simulink model "VelocityTransitionHandler"  (R2016b)
settings: Solver=FixedStepAuto  StartTime=0.0  StopTime=10.0  FixedStep=0.002  RelTol=1e-3  EnableMultiTasking=on
settings Model: Creator=march  LastModifiedBy=snyke7
settings SolverCC: EnableConcurrentExecution=on
settings DataIOCC: SaveFormat=StructureWithTime
settings OptimizationCC: BlockReduction=off  OptimizeBlockIOStorage=off  BufferReuse=off  GlobalBufferReuse=off  ExpressionFolding=off  LocalBlockOutputs=off
settings HardwareCC: ProdBitPerPointer=32  ProdBitPerSizeT=32  ProdBitPerPtrDiffT=32  ProdLargestAtomicFloat=None  ProdWordSize=32  ProdLongLongMode=on  ProdHWDeviceType=Generic->32-bit x86 compatible
settings RTWCC: SystemTargetFile=slrt.tlc  TemplateMakefile=slrt_default_tmf  Description=Simulink Real-Time  RTWCompilerOptimization=on
settings TargetCC: CodeReplacementLibrary=XPC_BLAS  ParMdlRefBuildCompliant=on  ConcurrentExecutionCompliant=on  GeneratePreprocessorConditionals=Use local settings  MatFileLogging=on  MATLABClassNameForMDSCustomization=xpcAperiodicCustomization

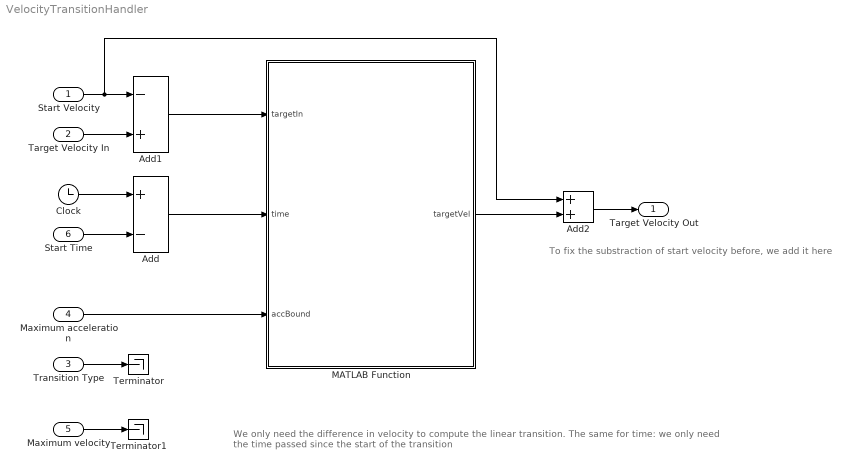
== system VelocityTransitionHandler ==
  note: To fix the substraction of start velocity before, we add it here
  note: We only need the difference in velocity to compute the linear transition. The same for time: we only need the time passed since the start of the transition
  Start Velocity : Inport
  Target Velocity In : Inport  Port=2
  Transition Type : Inport  Port=3
  Maximum acceleration : Inport  Port=4
  Maximum velocity : Inport  Port=5
  Start Time : Inport  Port=6
  Add : Sum  Inputs=+-
  Add1 : Sum  Inputs=-+
  Add2 : Sum
  Clock : Clock
  MATLAB Function : MATLAB Function  TreatAsAtomicUnit=on
  Terminator : Terminator
  Terminator1 : Terminator
  Target Velocity Out : Outport
  wires:
  Clock/1 -> Add/1
  Start Time/1 -> Add/2
  Start Velocity/1 -> Add2/1, Add1/1
  Target Velocity In/1 -> Add1/2
  Maximum velocity/1 -> Terminator1/1
  Transition Type/1 -> Terminator/1
  Add2/1 -> Target Velocity Out/1
  Add1/1 -> MATLAB Function/1(targetIn)
  Add/1 -> MATLAB Function/2(time)
  Maximum acceleration/1 -> MATLAB Function/3(accBound)
  MATLAB Function/1(targetVel) -> Add2/2

== matlab function VelocityTransitionHandler/MATLAB Function ==
  data: targetIn input; targetVel output; time input; accBound input
function targetVel = getTargetVelOut(targetIn, time, accBound)
%% GETTARGETVELOUT Calculates target velocity when transitioning to targetIn
% Calculates the target velocity at time time when transitioning linearly 
% with steepness accBound to targetIn

% v = at
targetVel = accBound * time;
if sign(targetIn) == -1
    % for negative targetpoints, v= -at
    targetVel = -1*targetVel;
end

% Once we have reached our target, stay at it
timeNeeded = abs(targetIn)/accBound;
if time > timeNeeded
    targetVel = targetIn;
end
end
